simulink model "statefdbk"  (R2015a)
settings: Solver=ode45  StartTime=0.0  StopTime=10.0  RelTol=1e-3
values from neighbouring files (symbols this model uses):
  C = eye(5)    [L6.m]
  D = [0 0 0 0 0]'    [L6.m]
  K = lqr(A, B, Qr, Rr)    [L6.m]
undefined symbols (not defined in the file or in its folder): A, B
settings Model: Creator=afons  LastModifiedBy=afons

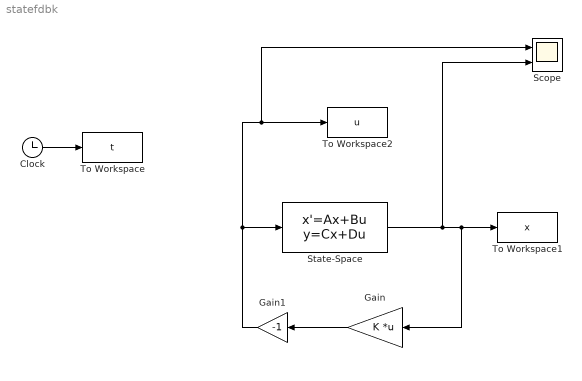
== system statefdbk ==
  Clock : Clock
  Gain : Gain  Gain=K  Multiplication=Matrix(K*u) (u vector)
  Gain1 : Gain  Gain=-1
  Scope : Scope  NumInputPorts=2
      settings: YMin=-5~-5  YMax=5~5
  State-Space : StateSpace  A=A  B=B  C=C  D=D  X0=5
  To Workspace : ToWorkspace  VariableName=t  SaveFormat=Timeseries  SampleTime=-1
  To Workspace1 : ToWorkspace  VariableName=x  SaveFormat=Timeseries  SampleTime=-1
  To Workspace2 : ToWorkspace  VariableName=u  SaveFormat=Timeseries  SampleTime=-1
  wires:
  Gain/1 -> Gain1/1
  State-Space/1 -> Scope/2, Gain/1, To Workspace1/1
  Gain1/1 -> Scope/1, To Workspace2/1, State-Space/1
  Clock/1 -> To Workspace/1
